simulink model "Hierarchy1NoActions"  (Simulink 9.0)
settings: Solver=ode3  StartTime=0.0  StopTime=10.0  RelTol=1e-3  EnableMultiTasking=on
settings Model: SuppressorTable=22 serialization::archive 11 0 6 0 0 0 0 0  Creator=scaife  LastModifiedBy=hbourbou  ExtModeAutoUpdateStatusClock=off
settings DataIOCC: LimitDataPoints=on  SignalLoggingSaveFormat=ModelDataLogs  SignalLoggingName=sigsOut
settings DebuggingCC: SaveWithParameterizedLinksMsg=none  SignalResolutionControl=TryResolveAllWithWarning  MultiTaskDSMMsg=warning  MultiTaskCondExecSysMsg=none  StrictBusMsg=None
settings HardwareCC: TargetUnknown=on
settings SFSimCC: SimParseCustomCode=off
settings GRTTargetCC: CombineOutputUpdateFcns=off  GRTInterface=on

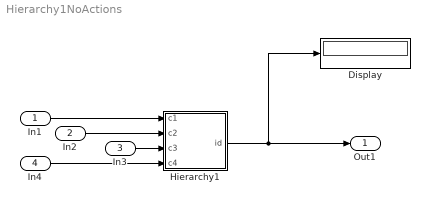
== system Hierarchy1NoActions ==
  In1 : Inport  OutDataTypeStr=boolean
  In2 : Inport  Port=2  OutDataTypeStr=boolean
  In3 : Inport  Port=3  OutDataTypeStr=boolean
  In4 : Inport  Port=4  OutDataTypeStr=boolean
  Display : Display
  Hierarchy1 : Stateflow chart  TreatAsAtomicUnit=on
  Out1 : Outport
  wires:
  Hierarchy1/1(id) -> Display/1, Out1/1
  In1/1 -> Hierarchy1/1(c1)
  In2/1 -> Hierarchy1/2(c2)
  In3/1 -> Hierarchy1/3(c3)
  In4/1 -> Hierarchy1/4(c4)

== stateflow chart Hierarchy1 ==
  state TOP/
    en:id=1;
    state N1/
      en:id=21;
      state A/
        en: id=31;
      state B/
        en: id=32;
      (default) -> A
      A -> B : [c4]
      B -> A : [c3]
    state N2/
      en:id=22;
      state C/
        en: id=33;
      state D/
        en: id=34;
      (default) -> C
      C -> D : [c4]
      D -> C : [c3]
    N2 -> N1 : [c1]
    (default) -> N1
    N1 -> N2 : [c2]
  (default) -> TOP
  data: c1 input double; c2 input double; c3 input double; c4 input double; id output double
